simulink model "podb"  (R2020a)
settings: Solver=ode45  StartTime=0.0  StopTime=500  RelTol=1e-3  EnableMultiTasking=on
values from neighbouring files (symbols this model uses):
  A1 = str2double(get(handles.edit5,'string'))    [Gui.m]
  A2 = str2double(get(handles.edit6,'string'))    [Gui.m]
  mi1 = str2double(get(handles.edit3,'string'))    [Gui.m]
  mi2 = str2double(get(handles.edit4,'string'))    [Gui.m]
  mu1 = str2double(get(handles.edit2,'string'))    [Gui.m]
settings Model: Creator=Sandra Knezevic  LastModifiedBy=Aldin
settings DataIOCC: LimitDataPoints=on  SaveFormat=Array  ReturnWorkspaceOutputs=off
settings OptimizationCC: LifeSpan=inf
settings DebuggingCC: SFUnexpectedBacktrackingDiag=warning  SFNoUnconditionalDefaultTransitionDiag=warning  SFExecutionAtInitializationDiag=none  ArithmeticOperatorsInVariantConditions=warning
settings HardwareCC: ProdBitPerPointer=32  ProdBitPerSizeT=32  ProdBitPerPtrDiffT=32  ProdLargestAtomicFloat=None  ProdIntDivRoundTo=Undefined  ProdEndianess=Unspecified  ProdWordSize=32  ProdHWDeviceType=32-bit Generic
settings ModelReferenceCC: PropagateSignalLabelsOutOfModel=off
settings SFSimCC: SimUseLocalCustomCode=off  CustomCodeUndefinedFunction=UseInterfaceOnly
settings RTWCC: RTWUseLocalCustomCode=off
settings CodeAppCC: StateflowObjectComments=on
settings GRTTargetCC: TargetLangStandard=C89/C90 (ANSI)
settings ConfigComp: CovMetricSettings=dw  CovHtmlReporting=on  CovSaveCumulativeToWorkspaceVar=on  CovSaveSingleToWorkspaceVar=on  CovExternalEMLEnable=off

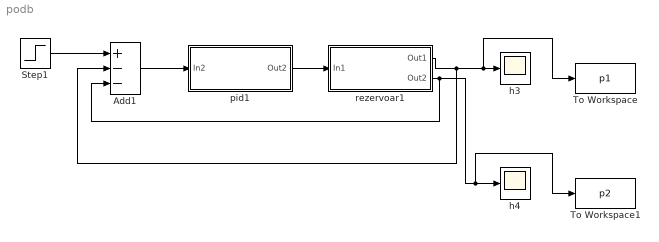
== system podb ==
  Add1 : Sum  Inputs=+--
  Step1 : Step  Time=0  Before=1  After=15  SampleTime=0
  To Workspace : ToWorkspace  VariableName=p1  SampleTime=-1
  To Workspace1 : ToWorkspace  VariableName=p2  SampleTime=-1
  h3 : Scope
  h4 : Scope
  pid1 : Subsystem
  rezervoar1 : Subsystem
  wires:
  pid1/1(Out2) -> rezervoar1/1(In1)
  Add1/1 -> pid1/1(In2)
  Step1/1 -> Add1/1
  rezervoar1/1(Out1) -> Add1/2, To Workspace/1, h3/1
  rezervoar1/2(Out2) -> Add1/3, To Workspace1/1, h4/1

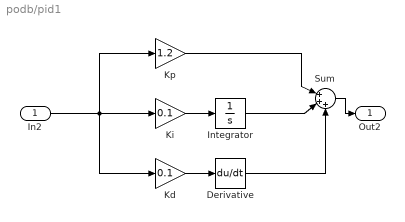
== system podb/pid1 ==
  In2 : Inport
  Derivative : Derivative
  Integrator : Integrator
  Kd : Gain  Gain=0.1
  Ki : Gain  Gain=0.1
  Kp : Gain  Gain=1.2
  Sum : Sum  Inputs=|+++
  Out2 : Outport
  wires:
  Kp/1 -> Sum/1
  Integrator/1 -> Sum/2
  Derivative/1 -> Sum/3
  Sum/1 -> Out2/1
  In2/1 -> Kp/1, Kd/1, Ki/1
  Ki/1 -> Integrator/1
  Kd/1 -> Derivative/1

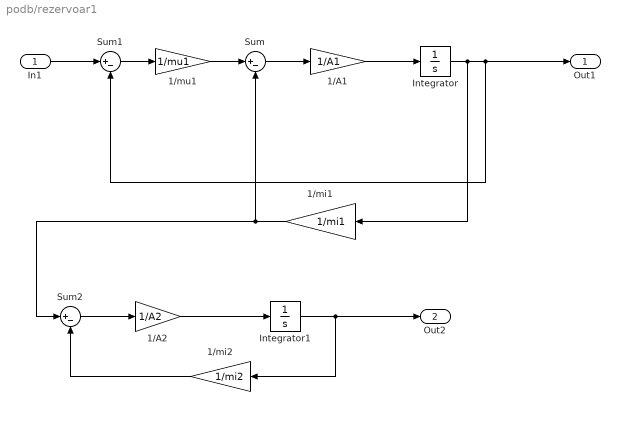
== system podb/rezervoar1 ==
  In1 : Inport
  1/A1 : Gain  Gain=1/A1
  1/A2 : Gain  Gain=1/A2
  1/mi1 : Gain  Gain=1/mi1
  1/mi2 : Gain  Gain=1/mi2
  1/mu1 : Gain  Gain=1/mu1
  Integrator : Integrator  InitialCondition=1
  Integrator1 : Integrator  InitialCondition=1
  Sum : Sum  Inputs=|+-
  Sum1 : Sum  Inputs=|+-
  Sum2 : Sum  Inputs=|+-
  Out1 : Outport
  Out2 : Outport  Port=2
  wires:
  1/A1/1 -> Integrator/1
  1/mu1/1 -> Sum/1
  Sum/1 -> 1/A1/1
  Sum1/1 -> 1/mu1/1
  In1/1 -> Sum1/1
  Integrator/1 -> 1/mi1/1, Sum1/2, Out1/1
  1/mi1/1 -> Sum/2, Sum2/1
  Sum2/1 -> 1/A2/1
  1/A2/1 -> Integrator1/1
  Integrator1/1 -> Out2/1, 1/mi2/1
  1/mi2/1 -> Sum2/2
